simulink model "Synchronous_Generators"  (R2025a)
settings: Solver=ode23tb  StartTime=0.0  StopTime=10.0  MaxStep=1e-4  RelTol=1e-3
libraries: spsSeriesRLCBranchLib x3, simulink x2, spsRMSLib x1, spsSynchronousMachinepuStandardLib x1, spsVoltageMeasurementLib x1, sps_lib x1
settings Model: Creator=Jawad  LastModifiedBy=Jawad

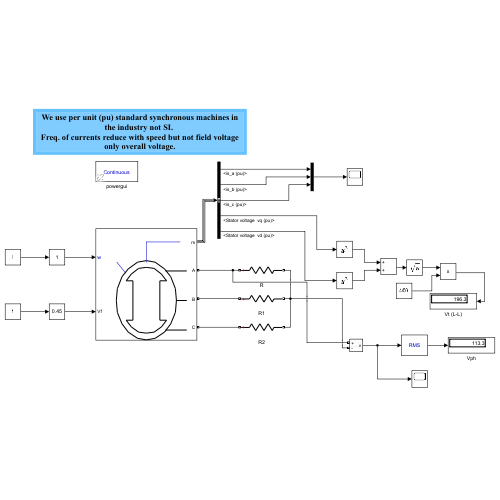
[thumbnail: Simulink's stored preview of the top-level diagram]
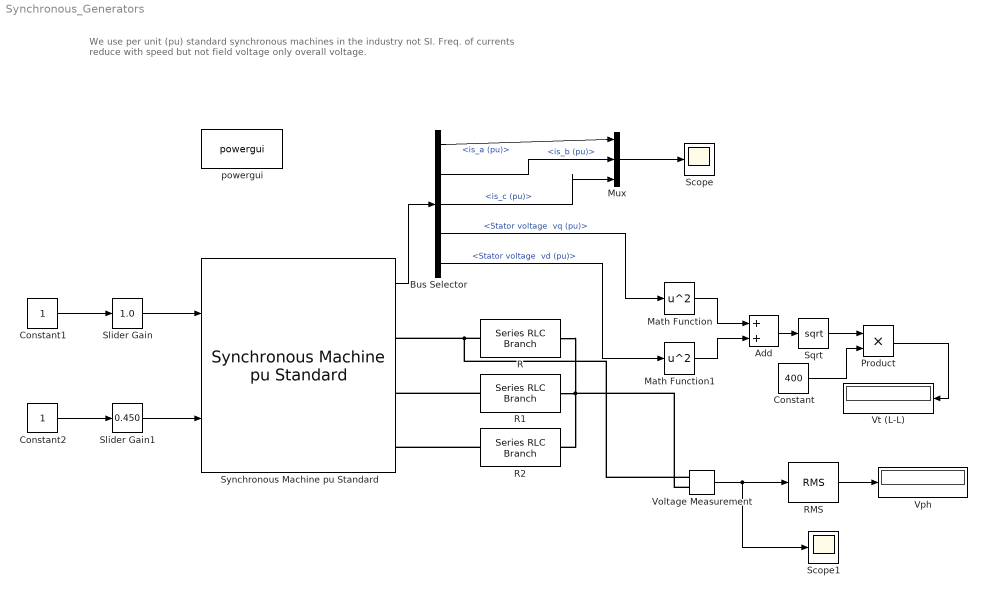
== system Synchronous_Generators ==
  note: We use per unit (pu) standard synchronous machines in the industry not SI.
      | Freq. of currents reduce with speed but not field voltage only overall voltage.
  Add : Sum
  Bus Selector : BusSelector  OutputSignals="Stator current.is_a (pu),Stator current.is_b (pu),Stator current.is_c (pu),dq0 components.Stator voltage  vq (pu),dq0 components.Stator voltage  vd (pu)"
  Constant : Constant  Value=400
  Constant1 : Constant
  Constant2 : Constant
  Math Function : Math  Operator=square
  Math Function1 : Math  Operator=square
  Mux : Mux  Inputs=3
  Product : Product
  R : spsSeriesRLCBranchLib/Series RLC Branch  LConnTagsString=__new0  RConnTagsString=__new0  BranchType=R  Resistance=100  Inductance=1e-3  SetiL0=off  InitialCurrent=0  Capacitance=1e-6  Setx0=off  InitialVoltage=0  Measurements=None
  R1 : spsSeriesRLCBranchLib/Series RLC Branch  LConnTagsString=__new0  RConnTagsString=__new0  BranchType=R  Resistance=100  Inductance=1e-3  SetiL0=off  InitialCurrent=0  Capacitance=1e-6  Setx0=off  InitialVoltage=0  Measurements=None
  R2 : spsSeriesRLCBranchLib/Series RLC Branch  LConnTagsString=__new0  RConnTagsString=__new0  BranchType=R  Resistance=100  Inductance=1e-3  SetiL0=off  InitialCurrent=0  Capacitance=1e-6  Setx0=off  InitialVoltage=0  Measurements=None
  RMS : spsRMSLib/RMS  TrueRMS=off  Freq=50  RMSInit=0  Ts=0
  Scope : Scope
      settings: ActiveDisplayYMinimum=-0.03604040331422529  ActiveDisplayYMaximum=0.036127724128330638
  Scope1 : Scope
      settings: ActiveDisplayYMinimum=-439.12589933871448  ActiveDisplayYMaximum=442.21943820321957
  Slider Gain : simulink/Math Operations/Slider Gain  gain=1.0  low=0  high=1
  Slider Gain1 : simulink/Math Operations/Slider Gain  gain=0.450  low=0  high=1
  Sqrt : Sqrt
  Synchronous Machine pu Standard : spsSynchronousMachinepuStandardLib/Synchronous Machine pu Standard  PresetModel=No  MechanicalLoad=Speed w  ShowDetailedParameters=on  RotorType=Salient-pole  Units=per unit standard parameters  MeasurementBus=off  NominalParameters=[6e+04 400 50]  Reactances1=[ 1.81, 0.3, 0.23, 1.76, 0.65, 0.25, 0.15 ]  Reactances2=[2.24 0.17 0.12 1.02 0.13 0.08]  dAxisTimeConstants=Short-circuit  qAxisTimeConstants=Short-circuit  TimeConstants1="[ 4.4849  0.0681  0.1  ]"  TimeConstants2=[ 8.0, 0.03, 1.0, 0.07 ]  TimeConstants3="[  4.49  0.0681  0.0513  ]"  TimeConstants4=[ 8.0, 0.03, 0.3371, 0.0295 ]  TimeConstants5=[ 1.01, 0.053, 0.1 ]  TimeConstants6=[ 1.3201, 0.023, 1.0, 0.07 ]  TimeConstants7=[0.012 0.003 0.003]  TimeConstants8=[ 1.3201, 0.0231, 0.3371, 0.0295 ]  StatorResistance=0.037875  Mechanical=[0.1028 0.02056 2]  PolePairs=20  InitialConditions="[ 0  0  0  0  0  0  0  0  1 ]"  SetSaturation=on  Saturation=[0.6404,0.7127,0.8441,0.9214,0.9956,1.082,1.19,1.316,1.457;0.7,0.7698,0.8872,0.9466,0.9969,1.046,1.1,1.151,1.201]  LoadFlowParameters=[1,0,0,0,0]  TsPowergui=0  TsBlock=-1  IterativeModel=Trapezoidal non iterative  IterativeDiscreteModel=Trapezoidal non iterative  BusType=PV  Pref=0  Qref=0  Qmin=-inf  Qmax=inf  PLF=0  QLF=0
  Voltage Measurement : spsVoltageMeasurementLib/Voltage Measurement  PhasorSimulation=off  OutputType=Complex  PSBequivalent=0
  Vph : Display
  Vt (L-L) : Display
  powergui : sps_lib/powergui  Priority=1  SimulationMode=Continuous  SampleTime=50e-6  frequency=60  Iterations=50  frequencyindice=50  Pbase=100e6  ErrMax=1e-4  UnitsV=kV  UnitsW=MW  buscounter=0  FunctionMessages=off  echomessages=off  EnableUseOfTLC=off  CurrentSourceSwitches=off  DisableSnubberDevices=off  DisableRonSwitches=off  DisableVfSwitches=off  DisplayEquations=off  AutomaticDiscreteSolvers=off  SolverType=Tustin/Backward Euler (TBE)  Interpol=off  ExternalGateDelay=off  methode=off  Ts=100  x0status=blocks  SPID=on  SwTol=0  HookPort=off  NonlinearTolerance=1e-4  nMaxIteration=100  ContinueOnMaxIteration=off  RestoreLinks=warning  ResistiveCurrentMeasurement=off  Frange=[0:2:500]  Ylog=off  Xlog=on  ShowGrid=off  save=off  variable=ZData  structure=0  ZoomFFT=off  StartTime=0.0  cycles=1  DisplayStyle=1  fundamental=60  FreqAxis=off  MaxFrequency=1000  frequencyindicesteady=1  RmsSteady=1  display=off
  wires:
  Synchronous Machine pu Standard/1 -> Bus Selector/1
  Bus Selector/1 -> Mux/1  "<is_a (pu)>"
  Bus Selector/2 -> Mux/2  "<is_b (pu)>"
  Bus Selector/3 -> Mux/3  "<is_c (pu)>"
  Bus Selector/4 -> Math Function/1  "<Stator voltage  vq (pu)>"
  Bus Selector/5 -> Math Function1/1  "<Stator voltage  vd (pu)>"
  Mux/1 -> Scope/1
  Math Function/1 -> Add/1
  Math Function1/1 -> Add/2
  Add/1 -> Sqrt/1
  Sqrt/1 -> Product/1
  Constant/1 -> Product/2
  Product/1 -> Vt (L-L)/1
  Voltage Measurement/1 -> Scope1/1, RMS/1
  RMS/1 -> Vph/1
  Constant1/1 -> Slider Gain/1
  Slider Gain/1 -> Synchronous Machine pu Standard/1
  Constant2/1 -> Slider Gain1/1
  Slider Gain1/1 -> Synchronous Machine pu Standard/2
  connections:
  R1/RConn1 -- R2/RConn1 -- Voltage Measurement/LConn2 -- R/RConn1
  R/LConn1 -- Voltage Measurement/LConn1 -- Synchronous Machine pu Standard/RConn1
  R1/LConn1 -- Synchronous Machine pu Standard/RConn2
  R2/LConn1 -- Synchronous Machine pu Standard/RConn3
